simulink model "ModelScheme_version2022"  (R2022b)
settings: Solver=VariableStepAuto  StartTime=0.0  StopTime=10  RelTol=1e-5
undefined symbols (not defined in the file or in its folder): A, d, D_C1, D_C2, D_C3, N_C1, N_C2, N_C3, P_l, P_r, r, Ts, Vbat, w_ref
settings Model: Creator=giorgia  LastModifiedBy=loren

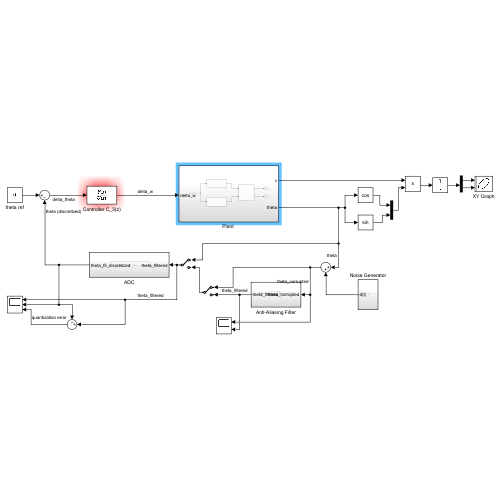
[thumbnail: Simulink's stored preview of the top-level diagram]
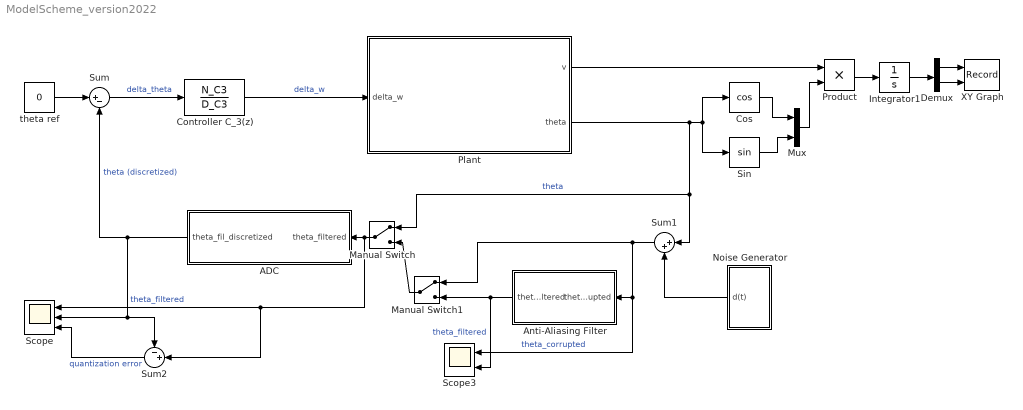
== system ModelScheme_version2022 ==
  ADC : Subsystem
  Anti-Aliasing Filter : Subsystem
  Controller C_3(z) : DiscreteTransferFcn  Numerator=N_C3  Denominator=D_C3
  Cos : Trigonometry  Operator=cos
  Demux : Demux  Outputs=2
  Integrator1 : Integrator
  Manual Switch : ManualSwitch
  Manual Switch1 : ManualSwitch
  Mux : Mux  Inputs=2
  Noise Generator : Subsystem
  "Plant " : Subsystem
  Product : Product
  Scope : Scope  NumInputPorts=3
  Scope3 : Scope  NumInputPorts=2
  Sin : Trigonometry
  Sum : Sum  Inputs=|+-
  Sum1 : Sum  Inputs=|++
  Sum2 : Sum  Inputs=-+|
  XY Graph : Record  FileSettingsInternal="{\"entries\":[{\"content\":{\"excelSettings\":{\"content\":{},\"type\":\"Streamout.ExcelSettings\"}},\"type\":\"Streamout.FileSettingStorage\",\"uuid\":\"\"}],\"packageUris\":[\"http:\\/\\/schema.mathworks.com\\/mf0\\/streamout_blocks\\/R2020a\"],\"version\":\"1.0\"}"  Layout=[1 1]  SignalsInternal="{\"entries\":[{\"content\":{\"signals\":[{\"content\":{\"blockPath\":[],\"channel\":[],\"dimensions\":[1],\"domain\":\"\",\"lineColor\":\"#a2142f\",\"plots\":[1],\"port\":1,\"sid\":[],\"signalID\":8,\"signalName\":\"Demux:1\"},\"type\":\"RecordBlkView.Signal\",\"uuid\":\"\"},{\"content\":{\"blockPath\":[],\"channel\":[],\"dimensions\":[1],\"domain\":\"\",\"lineColor\":\"#139fff\",\"plots\":[1],\"port\":2,\"sid\":[],\"signalID\":11,\"signalName\":\"Demux:2\"},\"type\":\"RecordBlkView.Signal\",\"uuid\":\"\"}]},\"type\":\"RecordBlkView.InputSignals\",\"uuid\":\"\"}],\"packageUris\":[\"http:\\/\\/schema.mathworks.com\\/mf0\\/streamout_blocks\\/R2020a\"],\"version\":\"1.0\"}"  VisualizationBindings="{\"xyplotplugin\":{\"info\":[{\"series\":[{\"bindingParametersList\":[{\"parameter\":\"X-Axis\",\"signalID\":8,\"signalName\":\"Demux:1\"},{\"parameter\":\"Y-Axis\",\"signalID\":11,\"signalName\":\"Demux:2\"}],\"seriesID\":11008}],\"subplotID\":1}]}}"  CompatibilityTag=XY
  theta ref : Constant  Value=0  SampleTime=Ts
  wires:
  Mux/1 -> Product/2
  Product/1 -> Integrator1/1
  Demux/2 -> XY Graph/2
  Demux/1 -> XY Graph/1
  Integrator1/1 -> Demux/1
  Sin/1 -> Mux/2
  Cos/1 -> Mux/1
  theta ref/1 -> Sum/1
  ADC/1(theta_fil_discretized) -> Sum2/1, Scope/2, Sum/2  "theta (discretized)"
  Sum/1 -> Controller C_3(z)/1  "delta_theta"
  Sum1/1 -> Scope3/1, Anti-Aliasing Filter/1(theta_corrupted), Manual Switch1/1  "theta_corrupted"
  "Plant "/2(theta) -> Manual Switch/1, Sum1/1, Sin/1, Cos/1  "theta"
  Controller C_3(z)/1 -> "Plant "/1(delta_w)  "delta_w"
  "Plant "/1(v) -> Product/1
  Sum2/1 -> Scope/3  "quantization error"
  Manual Switch/1 -> Sum2/2, Scope/1, ADC/1(theta_filtered)  "theta_filtered"
  Anti-Aliasing Filter/1(theta_filtered) -> Scope3/2, Manual Switch1/2  "theta_filtered"
  Manual Switch1/1 -> Manual Switch/2
  Noise Generator/1(d(t)) -> Sum1/2

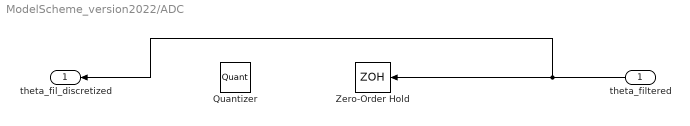
== system ModelScheme_version2022/ADC ==
  theta_filtered : Inport
  Quantizer : Quantizer  QuantizationInterval=delta_q3
  Zero-Order Hold : ZeroOrderHold  SampleTime=Ts
  theta_fil_discretized : Outport
  wires:
  theta_filtered/1 -> theta_fil_discretized/1, Zero-Order Hold/1

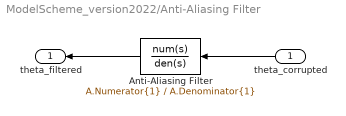
== system ModelScheme_version2022/Anti-Aliasing Filter ==
  theta_corrupted : Inport
  Anti-Aliasing Filter : TransferFcn  Numerator=A.Numerator{1}  Denominator=A.Denominator{1}
  theta_filtered : Outport
  wires:
  theta_corrupted/1 -> Anti-Aliasing Filter/1
  Anti-Aliasing Filter/1 -> theta_filtered/1

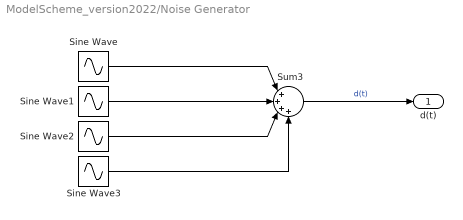
== system ModelScheme_version2022/Noise Generator ==
  Sine Wave : Sin  Frequency=5e5  SampleTime=0
  Sine Wave1 : Sin  Amplitude=2  Frequency=1e4  SampleTime=0
  Sine Wave2 : Sin  Amplitude=-1  Frequency=1e6  SampleTime=0
  Sine Wave3 : Sin  Amplitude=0.6  Frequency=6e3  SampleTime=0
  Sum3 : Sum  Inputs=|++++
  d(t) : Outport
  wires:
  Sum3/1 -> d(t)/1  "d(t)"
  Sine Wave1/1 -> Sum3/2
  Sine Wave/1 -> Sum3/1
  Sine Wave2/1 -> Sum3/3
  Sine Wave3/1 -> Sum3/4

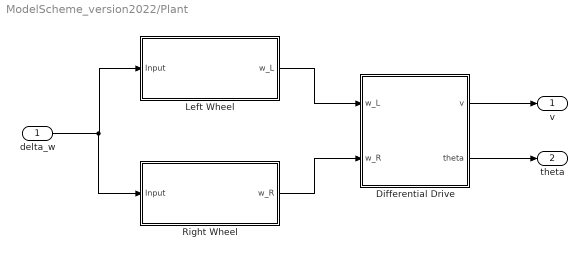
== system ModelScheme_version2022/Plant  ==
  delta_w : Inport
  Differential Drive : Subsystem
  Left Wheel : Subsystem
  Right Wheel : Subsystem
  v : Outport
  theta : Outport  Port=2
  wires:
  Differential Drive/1(v) -> v/1
  Right Wheel/1(w_R) -> Differential Drive/2(w_R)
  delta_w/1 -> Right Wheel/1(Input), Left Wheel/1(Input)
  Left Wheel/1(w_L) -> Differential Drive/1(w_L)
  Differential Drive/2(theta) -> theta/1

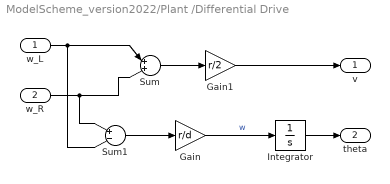
== system ModelScheme_version2022/Plant /Differential Drive ==
  w_L : Inport
  w_R : Inport  Port=2
  Gain : Gain  Gain=r/d
  Gain1 : Gain  Gain=r/2
  Integrator : Integrator  InitialCondition=pi/9
  Sum : Sum  Inputs=|++|
  Sum1 : Sum  Inputs=|+-|
  v : Outport
  theta : Outport  Port=2
  wires:
  w_L/1 -> Sum/1, Sum1/2
  w_R/1 -> Sum1/1, Sum/2
  Sum/1 -> Gain1/1
  Gain1/1 -> v/1
  Sum1/1 -> Gain/1
  Gain/1 -> Integrator/1  "w"
  Integrator/1 -> theta/1

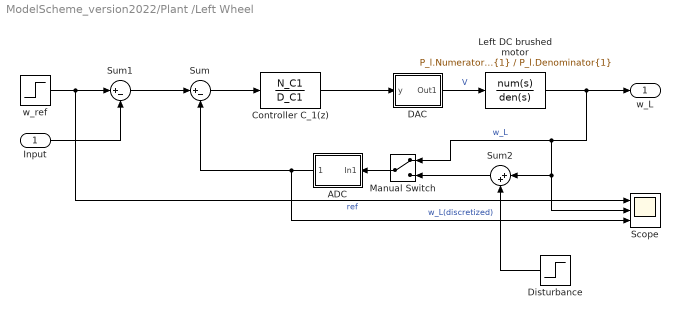
== system ModelScheme_version2022/Plant /Left Wheel ==
  Input : Inport
  ADC : Subsystem
  Controller C_1(z) : DiscreteTransferFcn  Numerator=N_C1  Denominator=D_C1
  DAC : Subsystem
  "Disturbance " : Step  Time=5  After=0.005  SampleTime=0
  Left DC brushed motor : TransferFcn  Numerator=P_l.Numerator{1}  Denominator=P_l.Denominator{1}
  Manual Switch : ManualSwitch
  Scope : Scope  NumInputPorts=3
  Sum : Sum  Inputs=|+-
  Sum1 : Sum  Inputs=|+-
  Sum2 : Sum  Inputs=|++
  w_ref : Step  After=w_ref  SampleTime=Ts
  w_L : Outport
  wires:
  DAC/1(Out1) -> Left DC brushed motor/1  "V"
  Left DC brushed motor/1 -> Manual Switch/1, Sum2/1, Scope/2, w_L/1  "w_L"
  w_ref/1 -> Scope/1, Sum1/1  "ref"
  Sum1/1 -> Sum/1
  Input/1 -> Sum1/2
  ADC/1(Out1) -> Scope/3, Sum/2  "w_L(discretized)"
  "Disturbance "/1 -> Sum2/2
  Manual Switch/1 -> ADC/1(In1)
  Sum2/1 -> Manual Switch/2
  Sum/1 -> Controller C_1(z)/1
  Controller C_1(z)/1 -> DAC/1(y)

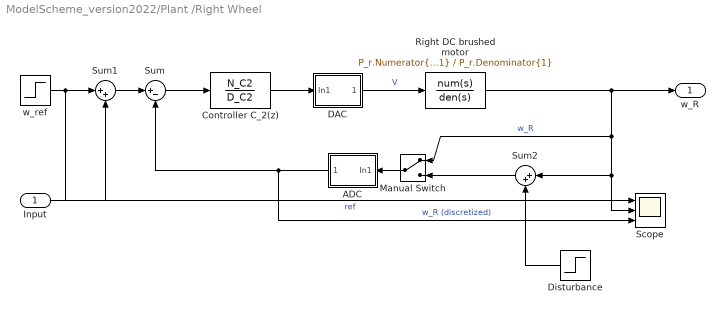
== system ModelScheme_version2022/Plant /Right Wheel ==
  Input : Inport
  ADC : Subsystem
  Controller C_2(z) : DiscreteTransferFcn  Numerator=N_C2  Denominator=D_C2
  DAC : Subsystem
  Disturbance : Step  Time=6  After=0.001  SampleTime=0
  Manual Switch : ManualSwitch
  Right DC brushed motor : TransferFcn  Numerator=P_r.Numerator{1}  Denominator=P_r.Denominator{1}
  Scope : Scope  NumInputPorts=3
  Sum : Sum  Inputs=|+-
  Sum1 : Sum  Inputs=|++
  Sum2 : Sum  Inputs=|++
  w_ref : Step  After=w_ref  SampleTime=Ts
  w_R : Outport
  wires:
  DAC/1(Out1) -> Right DC brushed motor/1  "V"
  Sum/1 -> Controller C_2(z)/1
  Right DC brushed motor/1 -> Scope/2, Sum2/1, Manual Switch/1, w_R/1  "w_R"
  Controller C_2(z)/1 -> DAC/1(In1)
  w_ref/1 -> Scope/1, Sum1/1  "ref"
  Sum1/1 -> Sum/1
  Input/1 -> Sum1/2
  ADC/1(Out1) -> Scope/3, Sum/2  "w_R (discretized)"
  Disturbance/1 -> Sum2/2
  Manual Switch/1 -> ADC/1(In1)
  Sum2/1 -> Manual Switch/2

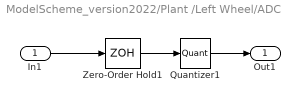
== system ModelScheme_version2022/Plant /Left Wheel/ADC ==
  In1 : Inport
  Quantizer1 : Quantizer  QuantizationInterval=delta_q2
  Zero-Order Hold1 : ZeroOrderHold  SampleTime=Ts
  Out1 : Outport
  wires:
  In1/1 -> Zero-Order Hold1/1
  Zero-Order Hold1/1 -> Quantizer1/1
  Quantizer1/1 -> Out1/1

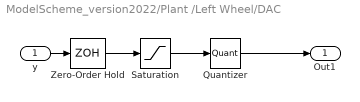
== system ModelScheme_version2022/Plant /Left Wheel/DAC ==
  y : Inport
  Quantizer : Quantizer  QuantizationInterval=delta_q1
  Saturation : Saturate  UpperLimit=Vbat  LowerLimit=-Vbat
  Zero-Order Hold : ZeroOrderHold  SampleTime=Ts
  Out1 : Outport
  wires:
  Quantizer/1 -> Out1/1
  Zero-Order Hold/1 -> Saturation/1
  y/1 -> Zero-Order Hold/1
  Saturation/1 -> Quantizer/1

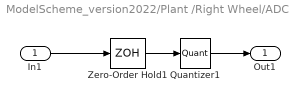
== system ModelScheme_version2022/Plant /Right Wheel/ADC ==
  In1 : Inport
  Quantizer1 : Quantizer  QuantizationInterval=delta_q2
  Zero-Order Hold1 : ZeroOrderHold  SampleTime=Ts
  Out1 : Outport
  wires:
  In1/1 -> Zero-Order Hold1/1
  Zero-Order Hold1/1 -> Quantizer1/1
  Quantizer1/1 -> Out1/1

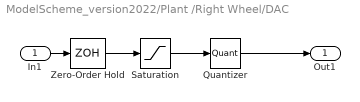
== system ModelScheme_version2022/Plant /Right Wheel/DAC ==
  In1 : Inport
  Quantizer : Quantizer  QuantizationInterval=delta_q1
  Saturation : Saturate  UpperLimit=Vbat  LowerLimit=-Vbat
  Zero-Order Hold : ZeroOrderHold  SampleTime=Ts
  Out1 : Outport
  wires:
  Quantizer/1 -> Out1/1
  Zero-Order Hold/1 -> Saturation/1
  In1/1 -> Zero-Order Hold/1
  Saturation/1 -> Quantizer/1
